simulink model "damped_systems"  (R2026a)
settings: Solver=VariableStepAuto  StopTime=20.0

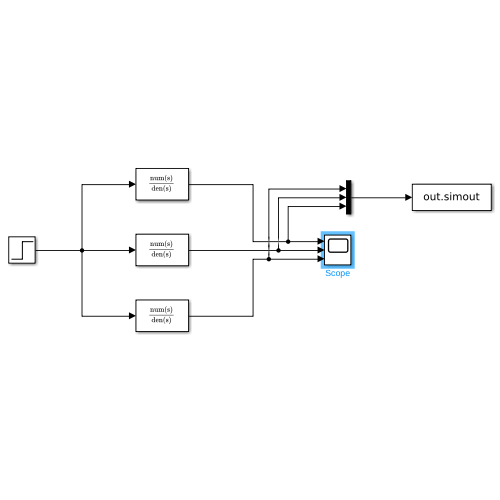
[thumbnail: Simulink's stored preview of the top-level diagram]
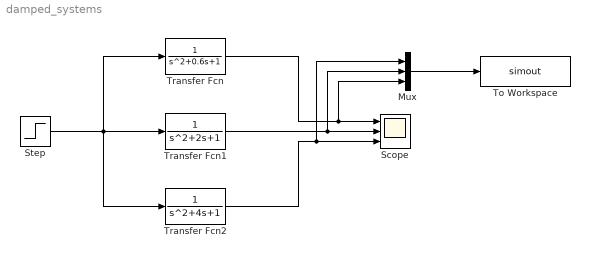
== system damped_systems ==
  Mux : Mux  Inputs=3
  Scope : Scope  NumInputPorts=3
      settings: ActiveDisplayYMinimum=-0.17153056921783683  ActiveDisplayYMaximum=1.5437751229605317
  Step : Step  SampleTime=0
  To Workspace : ToWorkspace  VariableName=simout  SaveFormat=Timeseries  SampleTime=-1
  Transfer Fcn : TransferFcn  Denominator=[1 0.6 1]
  Transfer Fcn1 : TransferFcn
  Transfer Fcn2 : TransferFcn  Denominator=[1 4 1]
  wires:
  Step/1 -> Transfer Fcn2/1, Transfer Fcn/1, Transfer Fcn1/1
  Mux/1 -> To Workspace/1
  Transfer Fcn/1 -> Mux/3, Scope/1
  Transfer Fcn1/1 -> Mux/2, Scope/2
  Transfer Fcn2/1 -> Mux/1, Scope/3
